simulink model "Single_motor_flyer_controller"  (R2018a)
settings: Solver=FixedStepAuto  StartTime=0.0  StopTime=10  FixedStep=0.01  RelTol=1e-3
libraries: dspindex x9
settings Model: Creator=WEIDONG  LastModifiedBy=dongw

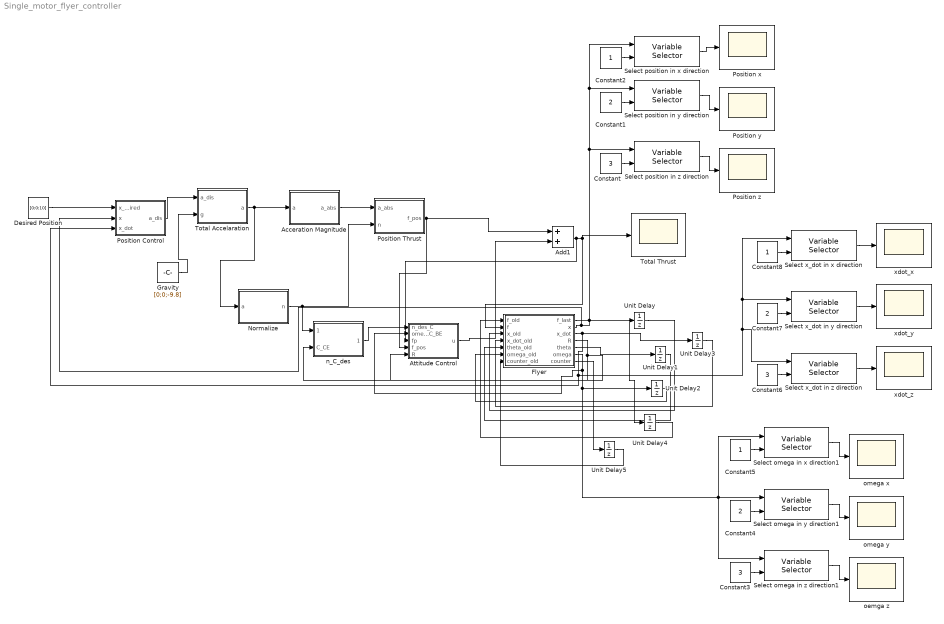
== system Single_motor_flyer_controller ==
  " Attitude Control" : MATLAB Function  TreatAsAtomicUnit=on
  Acceration Magnitude : MATLAB Function  TreatAsAtomicUnit=on
  Add1 : Sum
  Constant : Constant  Value=3
  Constant1 : Constant  Value=2
  Constant2 : Constant
  Constant3 : Constant  Value=3
  Constant4 : Constant  Value=2
  Constant5 : Constant
  Constant6 : Constant  Value=3
  Constant7 : Constant  Value=2
  Constant8 : Constant
  Desired Position : Constant  Value=[0;0;10]
  Flyer : MATLAB Function  TreatAsAtomicUnit=on
  Gravity : Constant  Value=[0;0;-9.8]
  Normalize : MATLAB Function  TreatAsAtomicUnit=on
  Position Control : MATLAB Function  TreatAsAtomicUnit=on
  Position Thrust : MATLAB Function  TreatAsAtomicUnit=on
  Position x : Scope
  Position y : Scope
  Position z : Scope
  Select omega in x direction1 : dspindex/Variable Selector  NumInputs=1  rowsOrCols=Rows  IdxMode=Variable  Elements=[1 3]  ZerOneIdxMode=One-based  errmode=Clip Index  FillMode=on  FillValues=0
  Select omega in y direction1 : dspindex/Variable Selector  NumInputs=1  rowsOrCols=Rows  IdxMode=Variable  Elements=[1 3]  ZerOneIdxMode=One-based  errmode=Clip Index  FillMode=on  FillValues=0
  Select omega in z direction1 : dspindex/Variable Selector  NumInputs=1  rowsOrCols=Rows  IdxMode=Variable  Elements=[1 3]  ZerOneIdxMode=One-based  errmode=Clip Index  FillMode=on  FillValues=0
  Select position in x direction : dspindex/Variable Selector  NumInputs=1  rowsOrCols=Rows  IdxMode=Variable  Elements=[1 3]  ZerOneIdxMode=One-based  errmode=Clip Index  FillMode=on  FillValues=0
  Select position in y direction : dspindex/Variable Selector  NumInputs=1  rowsOrCols=Rows  IdxMode=Variable  Elements=[1 3]  ZerOneIdxMode=One-based  errmode=Clip Index  FillMode=on  FillValues=0
  Select position in z direction : dspindex/Variable Selector  NumInputs=1  rowsOrCols=Rows  IdxMode=Variable  Elements=[1 3]  ZerOneIdxMode=One-based  errmode=Clip Index  FillMode=on  FillValues=0
  Select x_dot in x direction : dspindex/Variable Selector  NumInputs=1  rowsOrCols=Rows  IdxMode=Variable  Elements=[1 3]  ZerOneIdxMode=One-based  errmode=Clip Index  FillMode=on  FillValues=0
  Select x_dot in y direction : dspindex/Variable Selector  NumInputs=1  rowsOrCols=Rows  IdxMode=Variable  Elements=[1 3]  ZerOneIdxMode=One-based  errmode=Clip Index  FillMode=on  FillValues=0
  Select x_dot in z direction : dspindex/Variable Selector  NumInputs=1  rowsOrCols=Rows  IdxMode=Variable  Elements=[1 3]  ZerOneIdxMode=One-based  errmode=Clip Index  FillMode=on  FillValues=0
  Total Accelaration : MATLAB Function  TreatAsAtomicUnit=on
  Total Thrust : Scope
  Unit Delay{,1..5} (6 alike) : UnitDelay  SampleTime=-1
  n_C_des : MATLAB Function  TreatAsAtomicUnit=on
  oemga z : Scope
  omega x : Scope
  omega y : Scope
  xdot_x : Scope
  xdot_y : Scope
  xdot_z : Scope
  wires:
  Position Control/1(a_dis) -> Total Accelaration/1(a_dis)
  Flyer/3(x_dot) -> Select x_dot in z direction/1, Select x_dot in x direction/1, Select x_dot in y direction/1, Position Control/3(x_dot), Unit Delay3/1
  Gravity/1 -> Total Accelaration/2(g)
  Normalize/1(n) -> n_C_des/1(n_E_des), Position Thrust/2(n)
  Flyer/4(R) -> " Attitude Control"/5(R), n_C_des/2(C_CE)
  n_C_des/1(n_C_des) -> " Attitude Control"/1(n_des_C)
  Position Thrust/1(f_pos) -> " Attitude Control"/4(f_pos), Add1/1
  " Attitude Control"/1(u) -> Add1/2
  Add1/1 -> " Attitude Control"/3(fp), Total Thrust/1, Flyer/2(f)
  Acceration Magnitude/1(a_abs) -> Position Thrust/1(a_abs)
  Unit Delay/1 -> Flyer/3(x_old)
  Unit Delay3/1 -> Flyer/4(x_dot_old)
  Flyer/5(theta) -> Unit Delay1/1
  Unit Delay1/1 -> Flyer/5(theta_old)
  Unit Delay2/1 -> Flyer/6(omega_old)
  Constant/1 -> Select position in z direction/2
  Select position in z direction/1 -> Position z/1
  Desired Position/1 -> Position Control/1(x_desired)
  Flyer/2(x) -> Position Control/2(x), Unit Delay/1, Select position in x direction/1, Select position in y direction/1, Select position in z direction/1
  Constant1/1 -> Select position in y direction/2
  Select position in y direction/1 -> Position y/1
  Constant2/1 -> Select position in x direction/2
  Select position in x direction/1 -> Position x/1
  Flyer/6(omega) -> Unit Delay2/1, Select omega in z direction1/1, Select omega in x direction1/1, Select omega in y direction1/1, " Attitude Control"/2(omega_C_BE)
  Constant3/1 -> Select omega in z direction1/2
  Select omega in z direction1/1 -> oemga z/1
  Select omega in x direction1/1 -> omega x/1
  Constant4/1 -> Select omega in y direction1/2
  Constant5/1 -> Select omega in x direction1/2
  Select omega in y direction1/1 -> omega y/1
  Constant8/1 -> Select x_dot in x direction/2
  Constant7/1 -> Select x_dot in y direction/2
  Select x_dot in x direction/1 -> xdot_x/1
  Select x_dot in z direction/1 -> xdot_z/1
  Constant6/1 -> Select x_dot in z direction/2
  Select x_dot in y direction/1 -> xdot_y/1
  Flyer/1(f_last) -> Unit Delay4/1
  Unit Delay4/1 -> Flyer/1(f_old)
  Flyer/7(counter) -> Unit Delay5/1
  Unit Delay5/1 -> Flyer/7(counter_old)
  Total Accelaration/1(a) -> Acceration Magnitude/1(a), Normalize/1(a)

== matlab function Single_motor_flyer_controller/Position Control ==
  data: x_desired input; x input; a_dis output size=[3 1]; x_dot input
function a_dis = fcn(x_desired,x,x_dot)
    epsilon=1;
    omega=1;
    a_dis = -2*epsilon*omega.*x_dot-omega^2.*(x-x_desired);
end

== matlab function Single_motor_flyer_controller/Position Thrust ==
  data: a_abs input size=[1 1]; f_pos output; n input size=[3 1]
function f_pos = fcn(a_abs,n)
z_B=[0;0;1];
m=0.217;
if a_abs*m/dot(z_B,n)==0
    f_pos = 0;
else
    f_pos = a_abs*m/dot(z_B,n);
end
% f_p=0;

== matlab function Single_motor_flyer_controller/ Attitude Control ==
  data: n_des_C input size=[3 1]; u output; omega_C_BE input size=[3 1]; fp input; f_pos input; R input
function u = fcn(n_des_C,omega_C_BE,fp,f_pos,R)

    %Hover_solution
    omega_hover=[7.0;-3.7;22.4];
    fp_hover=2.26;
    %f_pos should not be one of the inputs
    %parameters
    g = [0; 0; -9.8];
    m = 0.5;
    d = [0.17,0,0];
    %Moment of Inertia
    I_B_B = diag([2.7*10e-3, 2.7*10e-3,5.2*10e-3]);  % Body Inertia
    I_B_P = diag([0, 0,1.5*10e-5]);  % Propeller Inertia
    %thrust and torque coefficient
    K_f=6.41*10^(-6);
    K_t=1.1 * 10^(-7);
    dt=0.01;%simulation time interval in seconds
    %drag coefficient
    K_B_d=diag([0.7*10e-4, 0.7*10e-4, 1.4*10e-4]);
    %s_dot1, s_dot2
    %S=[n_des_C(1,1),;n_des_C(2,1);omega_C_BE(1,1);omega_C_BE(2,1);omega_C_BE(3,1)];
    S=sym('S',[6 1]); %state
    
    syms u_sym %input
    n_des_C_sym=zeros(3,1);
    n_des_C_sym(1:2,1)=S(1:2,1);
    n_des_C_sym(3,1)=sqrt(1-S(1,1)^2-S(2,1)^2);
    omega_sym=S(3:5,1)-omega_hover;
    fp_sym=S(6,1)+fp_hover;
    n_des_C_dot=-cross(omega_sym,n_des_C_sym);
    fp_dot=(f_pos+u_sym-fp)/dt;
    
    %disregard drag and angular acceleration of the propeller, and
    %represent the thrust in the inertial frame in order to calculate the
    %angular acceleration of body in the inertial frame
    prop_speed_sq=fp_sym/K_f;
    prop_speed=[0;0;sqrt(abs(prop_speed_sq))];
    
    %From fp_dot=2*K_f*prop_speed_z*prop_speed_z_dot  (prop_speed_z is the scalar value of prop_speed)
    prop_ang_acc=[0;0;fp_dot/(2*K_f*sqrt(abs(prop_speed_sq))); 
    t_B_d=-sqrt(sum((omega_sym).^2))*K_B_d*omega_sym;
    T_p = [0;0;-prop_speed_sq* K_t];
    f_vector=[0; 0; -fp];
    tau=R*(cross(d',f_vector)+T_p);%total torque
    
    % omega_B_BE_dot
    omegadot = I_B_B\ (tau + t_B_d - cross(omega_sym, I_B_B * omega_sym+I_B_P*(R*prop_speed))-I_B_P*(R*prop_ang_acc));
    %S_dot
    S_dot=[n_des_C_dot(1:2,1);omegadot;fp_dot];
    %Jacobian
    A=jacobian(S_dot,S);
    B=jacobian(S_dot,[0;0;0;0;0;u_syms]);
    subs(A,S,zeros(6,1));
    subs(B,u_sym,fp_hover);
    %LQR
    Q=[75;75;0;0;0;0];
    R=zeros(6,1);
    N=zeros(6,1);
    [K,S,e] = LQR(A,B,Q,R,N);
    s=zeros(6,1);
    s(1:2,1)=n_des_C_sym(1:2,1);
    s(3:5,1)=omega_C_BE+omega_hover;
    s(6,1)=fp_sym-fp_hover;
    u = -K*s;
end

== matlab function Single_motor_flyer_controller/Flyer ==
  data: f_old input; f_last output; f input size=[1 1]; x_old input size=[3 1]; x_dot_old input size=[3 1]; x output size=[3 1]; x_dot output size=[3 1]; R output size=[3 3]; theta output size=[3 1]; theta_old input size=[3 1]; omega_old input size=[3 1]; omega output size=[3 1]; counter output; counter_old input
 function [f_last,x,x_dot,R,theta,omega,counter] = fcn(f_old,f,x_old,x_dot_old,theta_old,omega_old,counter_old)
% the block is based on the dynamics of a quadcopter on
% http://andrew.gibiansky.com/blog/physics/quadcopter-dynamics/
    counter=counter_old+1;
    
%Assume a friction coeffiicent
    kd=0.25;
    %initial states
    %row, pitch and yaw
    %theta = zeros(3,1);
    %thetadot = zeros(3,1);

    %parameters
    g = [0; 0; -9.8];
    m = 0.5;
    d = [0.17,0,0];

    I_B_B = diag([2.7*10e-3, 2.7*10e-3,5.2*10e-3]);  % Body Inertia
    I_B_P = diag([0, 0,1.5*10e-5]);  % Propeller Inertia
    %thrust and torque coefficient
    K_f=6.41*10^(-6);
    K_t=1.1 * 10^(-7);
    dt=0.01;%simulation time interval in seconds

    %aerodynamic drag torque
    K_B_d=diag([0.7*10e-4, 0.7*10e-4, 1.4*10e-4]);

    % Compute thrust given current inputs and thrust coefficient.
    %f = [0; 0; 6.41*10^(-6) * input*input];
    prop_speed_sq=f/K_f;
    prop_speed=[0;0;sqrt(abs(prop_speed_sq))];
    prop_speed_sq_old=f_old/K_f;
    prop_speed_old=[0;0;sqrt(abs(prop_speed_sq_old))];
    
    % Compute forces, torques, and accelerations.
    %omega = thetadot2omega(thetadot, theta);
    
    %rotation matrix from body frame to earth frame
    R = rotation(theta_old);
    %R=zeros(3,3);
    % Compute reaction torque, given current inputs, length, drag coefficient, and thrust coefficient.
    T_p = [0;0;-prop_speed_sq* K_t];
    f_vector=[0; 0; -f];
    T = R * f_vector;
    a = g + 1 / m .* T-kd*x_dot_old;
    %omegadot
    t_B_d=-sqrt(sum((omega_old).^2))*K_B_d*omega_old;
    
    tau=R*(cross(d',f_vector)+T_p);%total torque
    prop_ang_acc=(prop_speed-prop_speed_old)/dt;
    %prop_ang_acc=[0;0;0];
    %Main structure
    %omega_old = thetadot2omega(thetadot, theta);
    
    omegadot = I_B_B\ (tau + t_B_d - cross(omega_old, I_B_B * omega_old+I_B_P*(R*prop_speed))-I_B_P*(R*prop_ang_acc));
    if max(omegadot)>10^20
        omegadot=[0;0;0];
    end
    % Advance system state
    omega = omega_old + dt * omegadot;
    %omega=[0;0;0];
    thetadot = omega2thetadot(omega, theta_old); 
    theta = theta_old + dt * thetadot;
    x_dot = x_dot_old + a * dt;
    %x_dot=[0;0;0];
    x = x_old + dt * x_dot;
    f_last=f;
    %x=[0;0;0];
    %testing
    if counter==1000
        counter=1000;
    end
    if x_dot(3)<-10^3
        disp('J');
    end
end

== matlab function Single_motor_flyer_controller/n_C_des ==
  data: n_E_des input; n_C_des output; C_CE input size=[3,3]
function n_C_des = fcn(n_E_des,C_CE)

n_C_des=C_CE*n_E_des;

== matlab function Single_motor_flyer_controller/Acceration Magnitude ==
  data: a input size=[3 1]; a_abs output size=[1 1]
function a_abs = fcn(a)

a_abs = sqrt(abs(dot(a,a)));

== matlab function Single_motor_flyer_controller/Total Accelaration ==
  data: a_dis input size=[3 1]; a output size=[3 1]; g input size=[3 1]
function a = fcn(a_dis,g)

a=a_dis-g;

== matlab function Single_motor_flyer_controller/Normalize ==
  data: a input size=[3 1]; n output size=[3 1]
function n = fcn(a)
a_abs = sqrt(abs(dot(a,a)));
n=a/a_abs;
